simulink model "OpenEndWinding_base"  (R2023b)
settings: Solver=VariableStepAuto  StartTime=0.0  StopTime=0.2  RelTol=1e-3  AbsTol=1e-3  EnableMultiTasking=on
values from neighbouring files (symbols this model uses):
  FSW = 36000    [OpenEndWinding_sim.m]
  Ki = C.Ki    [OpenEndWinding_sim.m]
  Kp = C.Kp    [OpenEndWinding_sim.m]
  Rm = 10e-3    (= 0.01)    [OpenEndWinding_sim.m]
  sample_time = 1e-6    (= 1e-06)    [OpenEndWinding_sim.m]
libraries: ee_lib x24, nesl_utility x24, fl_lib x11, simulink x2, eeLCFB1 x1, slpidlib x1, spsTriangleGeneratorLib x1, spspowerguiLib x1
(part 2 of 2)

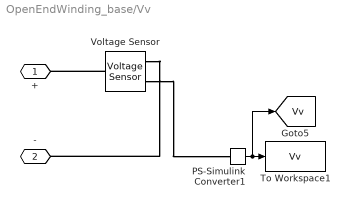
== system OpenEndWinding_base/Vv ==
  PS-Simulink Converter1 : nesl_utility/PS-Simulink Converter  PhysicalDomain=network_engine_domain  SubClassName=ps_output  LeftPortType=input  RightPortType=output  PseudoPeriodic=off  Frequencies=[]  VectorFormat=1-D array  Unit=V  AffineConversion=off
  To Workspace1 : ToWorkspace  VariableName=Vv  SampleTime=SampleTime
  Voltage Sensor : fl_lib/Electrical/Electrical Sensors/Voltage Sensor
  + : PMIOPort  Side=Left
  - : PMIOPort  Port=2  Side=Left
  tag scope: Vv=global
  wires:
  PS-Simulink Converter1/1 -> To Workspace1/1, [Vv]
  connections:
  Voltage Sensor/RConn1 -- PS-Simulink Converter1/LConn1
  Voltage Sensor/RConn2 -- -/RConn1
  Voltage Sensor/LConn1 -- +/RConn1

== system OpenEndWinding_base/Vw ==
  PS-Simulink Converter1 : nesl_utility/PS-Simulink Converter  PhysicalDomain=network_engine_domain  SubClassName=ps_output  LeftPortType=input  RightPortType=output  PseudoPeriodic=off  Frequencies=[]  VectorFormat=1-D array  Unit=V  AffineConversion=off
  To Workspace1 : ToWorkspace  VariableName=Vw  SampleTime=SampleTime
  Voltage Sensor : fl_lib/Electrical/Electrical Sensors/Voltage Sensor
  + : PMIOPort  Side=Left
  - : PMIOPort  Port=2  Side=Left
  tag scope: Vw=global
  wires:
  PS-Simulink Converter1/1 -> To Workspace1/1, [Vw]
  connections:
  Voltage Sensor/RConn1 -- PS-Simulink Converter1/LConn1
  Voltage Sensor/RConn2 -- -/RConn1
  Voltage Sensor/LConn1 -- +/RConn1

== system OpenEndWinding_base/TotemPole_SwitchMake/Subsystem ==
  Gain1 : Gain  Gain=1/2
  "Offset " : Constant
  Sum1 : Sum  Inputs=|++
  Triangle Generator1 : spsTriangleGeneratorLib/Triangle Generator  Freq=Freq  Phase=0  Ts=Ts
      settings: AttributesFormatString=Freq = %<Freq> Hz
  Out1 : Outport  VectorParamsAs1DForOutWhenUnconnected=off
  wires:
  "Offset "/1 -> Sum1/2
  Sum1/1 -> Gain1/1
  Gain1/1 -> Out1/1
  Triangle Generator1/1 -> Sum1/1
